simulink subsystem "SMC_mathmatical"  (R2023a)
settings: Solver=VariableStepAuto  StartTime=0.0  StopTime=10.0  RelTol=1e-3

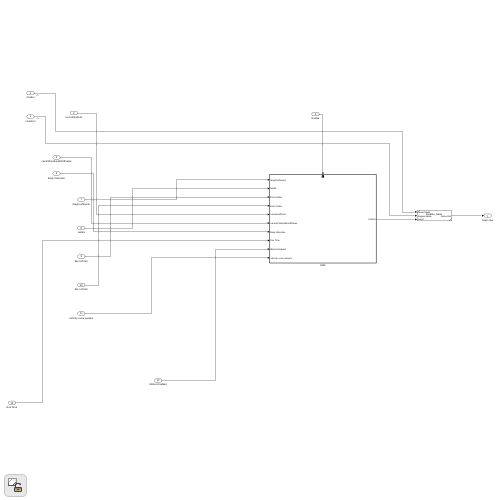
[thumbnail: Simulink's stored preview of the top-level diagram]
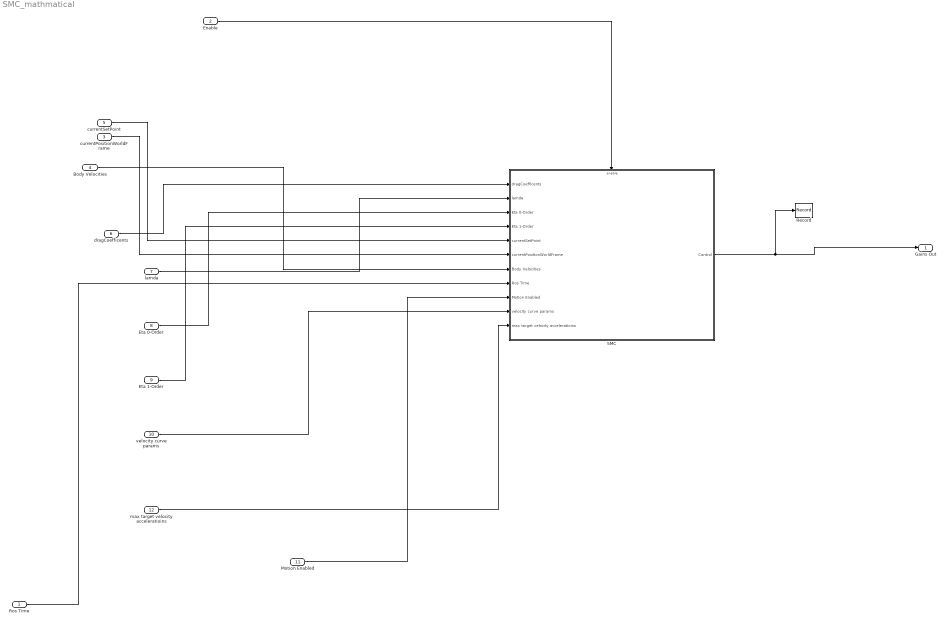
== system SMC_mathmatical ==
  Ros Time : Inport
  Enable : Inport  Port=2
  currentPositionWorldFrame : Inport  Port=3
  Body Velocities : Inport  Port=4
  currentSetPoint : Inport  Port=5
  dragCoefficents : Inport  Port=6
  lamda : Inport  Port=7
  Eta 0-Order : Inport  Port=8
  Eta 1-Order : Inport  Port=9
  velocity curve params : Inport  Port=10
  Motion Enabled : Inport  Port=11
  max target velocity acceleratioins : Inport  Port=12
  Record : Record  FileSettingsInternal="{\"entries\":[{\"content\":{\"excelSettings\":{\"content\":{},\"type\":\"Streamout.ExcelSettings\"}},\"type\":\"Streamout.FileSettingStorage\",\"uuid\":\"\"}],\"packageUris\":[\"http:\\/\\/schema.mathworks.com\\/mf0\\/streamout_blocks\\/R2020a\"],\"version\":\"1.0\"}"  Layout=[1 1]  SignalsInternal="{\"entries\":[{\"content\":{\"signals\":[{\"content\":{\"blockPath\":[],\"dimensions\":[6],\"domain\":\"\",\"hasChildren\":true,\"lineColor\":\"#22b573\",\"port\":1,\"signalID\":150872,\"signalName\":\"SMC\"},\"type\":\"RecordBlkView.Signal\",\"uuid\":\"\"},{\"content\":{\"blockPath\":[],\"channel\":[1],\"dimensions\":[6],\"domain\":\"\",\"lineColor\":\"#0072bd\",\"parentID\":150872,\"plots\":[1],\"port\":1,\"signalID\":150873,\"signalName\":\"SMC\"},\"type\":\"Rec ...(+1177 chars)"  VisualizationBindings="{\"sparklinesplugin\":{\"info\":[{\"bindingParametersList\":[],\"subplotID\":1}]}}"
  SMC : Subsystem
  Gains Out : Outport
  wires:
  SMC/1(Control) -> Gains Out/1, Record/1
  Eta 1-Order/1 -> SMC/4(Eta 1-Order)
  Body Velocities/1 -> SMC/7(Body Velocities)
  Motion Enabled/1 -> SMC/9(Motion Enabled)
  currentPositionWorldFrame/1 -> SMC/6(currentPositionWorldFrame)
  dragCoefficents/1 -> SMC/1(dragCoefficents)
  velocity curve params/1 -> SMC/10(velocity curve params)
  currentSetPoint/1 -> SMC/5(currentSetPoint)
  Enable/1 -> SMC/Enable
  Ros Time/1 -> SMC/8(Ros Time)
  lamda/1 -> SMC/2(lamda)
  Eta 0-Order/1 -> SMC/3(Eta 0-Order)
  max target velocity acceleratioins/1 -> SMC/11(max target velocity acceleratioins)

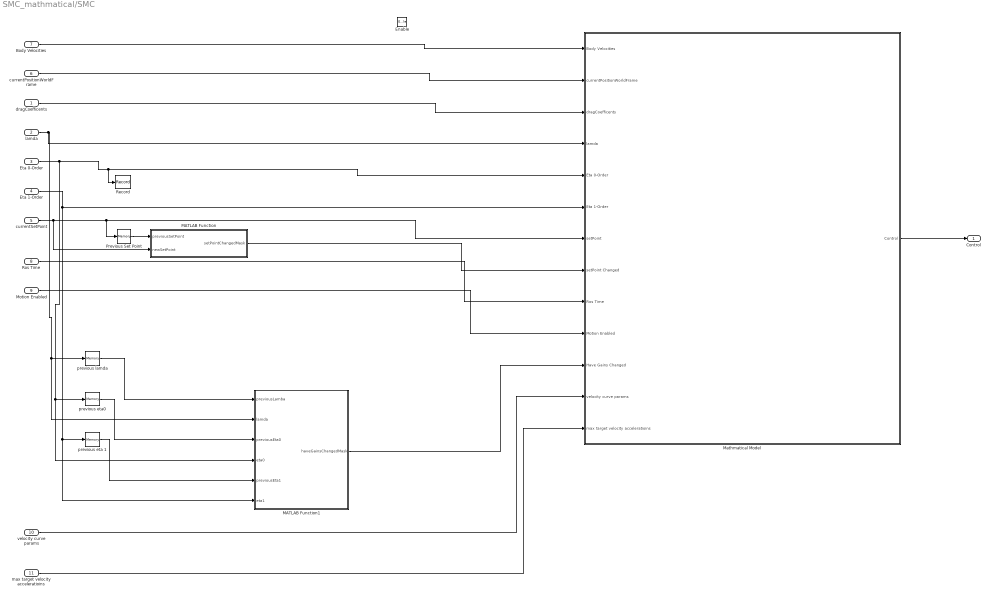
== system SMC_mathmatical/SMC ==
  dragCoefficents : Inport
  lamda : Inport  Port=2
  Eta 0-Order : Inport  Port=3
  Eta 1-Order : Inport  Port=4
  currentSetPoint : Inport  Port=5
  currentPositionWorldFrame : Inport  Port=6
  Body Velocities : Inport  Port=7
  Ros Time : Inport  Port=8
  Motion Enabled : Inport  Port=9
  velocity curve params : Inport  Port=10
  max target velocity acceleratioins : Inport  Port=11
  Enable : EnablePort
  MATLAB Function : MATLAB Function  TreatAsAtomicUnit=on
  MATLAB Function1 : MATLAB Function  TreatAsAtomicUnit=on
  Mathmatical Model : Subsystem
  Previous Set Point : Memory  InitialCondition=[0,0,0,0,0,0,0]  InheritSampleTime=on
  Record : Record  FileSettingsInternal="{\"entries\":[{\"content\":{\"excelSettings\":{\"content\":{},\"type\":\"Streamout.ExcelSettings\"}},\"type\":\"Streamout.FileSettingStorage\",\"uuid\":\"\"}],\"packageUris\":[\"http:\\/\\/schema.mathworks.com\\/mf0\\/streamout_blocks\\/R2020a\"],\"version\":\"1.0\"}"  Layout=[1 1]  SignalsInternal="{\"entries\":[{\"content\":{\"signals\":[{\"content\":{\"blockPath\":[],\"dimensions\":[1,6],\"domain\":\"\",\"hasChildren\":true,\"lineColor\":\"#139fff\",\"port\":1,\"signalID\":151262,\"signalName\":\"Eta 0-Order\"},\"type\":\"RecordBlkView.Signal\",\"uuid\":\"\"},{\"content\":{\"blockPath\":[],\"channel\":[1,1],\"dimensions\":[1,6],\"domain\":\"\",\"lineColor\":\"#edb120\",\"parentID\":151262,\"port\":1,\"signalID\":151263,\"signalName\":\"Eta 0-Order\"},\" ...(+1247 chars)"  VisualizationBindings="{\"sparklinesplugin\":{\"info\":[{\"bindingParametersList\":[],\"subplotID\":1}]}}"
  previous eta 1 : Memory  InheritSampleTime=on
  previous eta0 : Memory  InheritSampleTime=on
  previous lamda : Memory  InheritSampleTime=on
  Control : Outport
  wires:
  max target velocity acceleratioins/1 -> Mathmatical Model/13(max target velocity acceleratioins)
  velocity curve params/1 -> Mathmatical Model/12(velocity curve params)
  MATLAB Function1/1(haveGainsChangedMask) -> Mathmatical Model/11(Have Gains Changed)
  Eta 1-Order/1 -> Mathmatical Model/6(Eta 1-Order), MATLAB Function1/6(eta1), previous eta 1/1
  Eta 0-Order/1 -> MATLAB Function1/4(eta0), previous eta0/1, Mathmatical Model/5(Eta 0-Order), Record/1
  lamda/1 -> previous lamda/1, MATLAB Function1/2(lamda), Mathmatical Model/4(lamda)
  previous eta 1/1 -> MATLAB Function1/5(previousEta1)
  previous eta0/1 -> MATLAB Function1/3(previousEta0)
  previous lamda/1 -> MATLAB Function1/1(previousLamba)
  Motion Enabled/1 -> Mathmatical Model/10(Motion Enabled)
  Ros Time/1 -> Mathmatical Model/9(Ros Time)
  Previous Set Point/1 -> MATLAB Function/1(previousSetPoint)
  MATLAB Function/1(setPointChangedMask) -> Mathmatical Model/8(setPoint Changed)
  Body Velocities/1 -> Mathmatical Model/1(Body Velocities)
  currentPositionWorldFrame/1 -> Mathmatical Model/2(currentPositionWorldFrame)
  currentSetPoint/1 -> Mathmatical Model/7(setPoint), Previous Set Point/1, MATLAB Function/2(newSetPoint)
  Mathmatical Model/1(Control) -> Control/1
  dragCoefficents/1 -> Mathmatical Model/3(dragCoefficents)

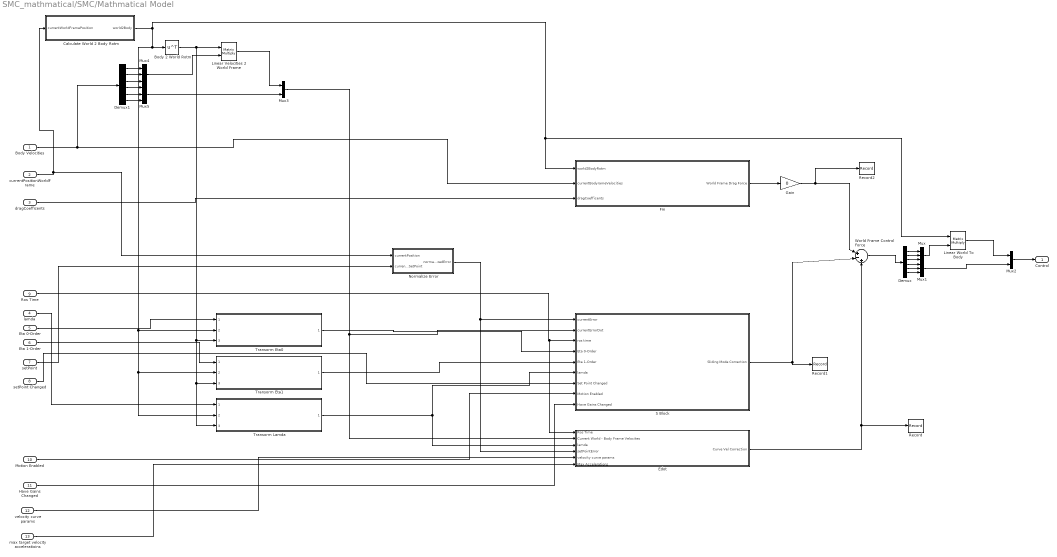
== system SMC_mathmatical/SMC/Mathmatical Model ==
  Body Velocities : Inport
  currentPositionWorldFrame : Inport  Port=2
  dragCoefficents : Inport  Port=3
  lamda : Inport  Port=4
  Eta 0-Order : Inport  Port=5
  Eta 1-Order : Inport  Port=6
  setPoint : Inport  Port=7
  setPoint Changed : Inport  Port=8
  Ros Time : Inport  Port=9
  Motion Enabled : Inport  Port=10
  Have Gains Changed : Inport  Port=11
  velocity curve params : Inport  Port=12
  max target velocity acceleratioins : Inport  Port=13
  Body 2 World Rotm : Math  Operator=transpose
  Calculate World 2 Body Rotm : MATLAB Function  TreatAsAtomicUnit=on
  Demux : Demux  Outputs=6
  Demux1 : Demux  Outputs=6
  Edot : Subsystem
  Fm : Subsystem
  Gain : Gain  Gain=0
  Linear Velocities 2 World Frame : Product  Multiplication=Matrix(*)
  Linear World To Body : Product  Multiplication=Matrix(*)
  Mux{,1,4..5} (4 alike) : Mux  Inputs=3
  Mux2 : Mux  Inputs=2
  Mux3 : Mux  Inputs=2
  Normalize Error : MATLAB Function  TreatAsAtomicUnit=on
  Record : Record  FileSettingsInternal="{\"entries\":[{\"content\":{\"excelSettings\":{\"content\":{},\"type\":\"Streamout.ExcelSettings\"}},\"type\":\"Streamout.FileSettingStorage\",\"uuid\":\"\"}],\"packageUris\":[\"http:\\/\\/schema.mathworks.com\\/mf0\\/streamout_blocks\\/R2020a\"],\"version\":\"1.0\"}"  Layout=[1 1]  SignalsInternal="{\"entries\":[{\"content\":{\"signals\":[{\"content\":{\"blockPath\":[],\"dimensions\":[6,1],\"domain\":\"\",\"hasChildren\":true,\"lineColor\":\"#ff6929\",\"port\":1,\"signalID\":150991,\"signalName\":\"Edot\"},\"type\":\"RecordBlkView.Signal\",\"uuid\":\"\"},{\"content\":{\"blockPath\":[],\"channel\":[1,1],\"dimensions\":[6,1],\"domain\":\"\",\"lineColor\":\"#4dbeee\",\"parentID\":150991,\"plots\":[1],\"port\":1,\"signalID\":150992,\"signalName\":\"Edot\"},\"ty ...(+1210 chars)"  VisualizationBindings="{\"sparklinesplugin\":{\"info\":[{\"bindingParametersList\":[],\"subplotID\":1}]}}"
  Record1 : Record  FileSettingsInternal="{\"entries\":[{\"content\":{\"excelSettings\":{\"content\":{},\"type\":\"Streamout.ExcelSettings\"}},\"type\":\"Streamout.FileSettingStorage\",\"uuid\":\"\"}],\"packageUris\":[\"http:\\/\\/schema.mathworks.com\\/mf0\\/streamout_blocks\\/R2020a\"],\"version\":\"1.0\"}"  Layout=[1 1]  SignalsInternal="{\"entries\":[{\"content\":{\"signals\":[{\"content\":{\"blockPath\":[],\"dimensions\":[6,1],\"domain\":\"\",\"hasChildren\":true,\"lineColor\":\"#fe330a\",\"port\":1,\"signalID\":151008,\"signalName\":\"S Block\"},\"type\":\"RecordBlkView.Signal\",\"uuid\":\"\"},{\"content\":{\"blockPath\":[],\"channel\":[1,1],\"dimensions\":[6,1],\"domain\":\"\",\"lineColor\":\"#0072bd\",\"parentID\":151008,\"plots\":[1],\"port\":1,\"signalID\":151009,\"signalName\":\"S Block ...(+1231 chars)"  VisualizationBindings="{\"sparklinesplugin\":{\"info\":[{\"bindingParametersList\":[],\"subplotID\":1}]}}"
  Record2 : Record  FileSettingsInternal="{\"entries\":[{\"content\":{\"excelSettings\":{\"content\":{},\"type\":\"Streamout.ExcelSettings\"}},\"type\":\"Streamout.FileSettingStorage\",\"uuid\":\"\"}],\"packageUris\":[\"http:\\/\\/schema.mathworks.com\\/mf0\\/streamout_blocks\\/R2020a\"],\"version\":\"1.0\"}"  Layout=[1 1]  SignalsInternal="{\"entries\":[{\"content\":{\"signals\":[{\"content\":{\"blockPath\":[],\"dimensions\":[6],\"domain\":\"\",\"hasChildren\":true,\"lineColor\":\"#22b573\",\"port\":1,\"signalID\":151025,\"signalName\":\"Gain\"},\"type\":\"RecordBlkView.Signal\",\"uuid\":\"\"},{\"content\":{\"blockPath\":[],\"channel\":[1],\"dimensions\":[6],\"domain\":\"\",\"lineColor\":\"#edb120\",\"parentID\":151025,\"plots\":[1],\"port\":1,\"signalID\":151026,\"signalName\":\"Gain\"},\"type\":\"R ...(+1232 chars)"  VisualizationBindings="{\"sparklinesplugin\":{\"info\":[{\"bindingParametersList\":[],\"subplotID\":1}]}}"
  S Block : Subsystem
  Transorm Eta0 : Subsystem  ReferencedSubsystem=Tranfsform_Linear_Gains_To_World
  Transorm Eta1 : Subsystem  ReferencedSubsystem=Tranfsform_Linear_Gains_To_World
  Transorm Lamda : Subsystem  ReferencedSubsystem=Tranfsform_Linear_Gains_To_World
  World Frame Control Force : Sum  Inputs=|+-+
  Control : Outport
  wires:
  max target velocity acceleratioins/1 -> Edot/6(Max Accelerations)
  velocity curve params/1 -> Edot/5(velocity curve params)
  Have Gains Changed/1 -> S Block/9(Have Gains Changed)
  Motion Enabled/1 -> S Block/8(Motion Enabled)
  Transorm Eta0/1 -> S Block/4(Eta 0-Order)
  Body 2 World Rotm/1 -> Linear Velocities 2 World Frame/1, Transorm Eta0/3, Transorm Eta1/3, Transorm Lamda/3
  Edot/1(Curve Vel Correction) -> World Frame Control Force/3, Record/1
  Gain/1 -> World Frame Control Force/1, Record2/1
  Eta 1-Order/1 -> Transorm Eta1/1
  setPoint/1 -> Normalize Error/2(currentSetPoint)
  Normalize Error/1(normalizedError) -> S Block/1(currentError), Edot/4(setPointError)
  Ros Time/1 -> S Block/3(ros time), Edot/1(Ros Time)
  setPoint Changed/1 -> S Block/7(Set Point Changed)
  Mux3/1 -> Edot/2(Current World - Body Frame Velocites), S Block/2(currentErrorDot)
  Eta 0-Order/1 -> Transorm Eta0/1
  lamda/1 -> Transorm Lamda/1
  Transorm Eta1/1 -> S Block/5(Eta 1-Order)
  Transorm Lamda/1 -> Edot/3(lamda), S Block/6(lamda)
  Mux5/1 -> Mux3/2
  Fm/1(World Frame Drag Force) -> Gain/1
  Demux1/6 -> Mux5/3
  Demux1/4 -> Mux5/1
  Demux1/5 -> Mux5/2
  Demux1/3 -> Mux4/3
  Demux1/1 -> Mux4/1
  Demux1/2 -> Mux4/2
  Mux4/1 -> Linear Velocities 2 World Frame/2
  Linear Velocities 2 World Frame/1 -> Mux3/1
  dragCoefficents/1 -> Fm/3(dragCoefficents)
  Calculate World 2 Body Rotm/1(world2Body) -> Fm/1(world2BodyRotm), Linear World To Body/1, Transorm Lamda/2, Transorm Eta1/2, Transorm Eta0/2, Body 2 World Rotm/1
  Mux2/1 -> Control/1
  Mux1/1 -> Mux2/2
  Linear World To Body/1 -> Mux2/1
  Mux/1 -> Linear World To Body/2
  Demux/4 -> Mux1/1
  Demux/5 -> Mux1/2
  Demux/6 -> Mux1/3
  Demux/3 -> Mux/3
  Demux/2 -> Mux/2
  Demux/1 -> Mux/1
  World Frame Control Force/1 -> Demux/1
  S Block/1("Sliding Mode Correction ") -> Record1/1, World Frame Control Force/2
  currentPositionWorldFrame/1 -> Calculate World 2 Body Rotm/1(currentWorldFramePosition), Normalize Error/1(currentPosition)
  Body Velocities/1 -> Demux1/1, Fm/2(currentBodyrameVelocities)

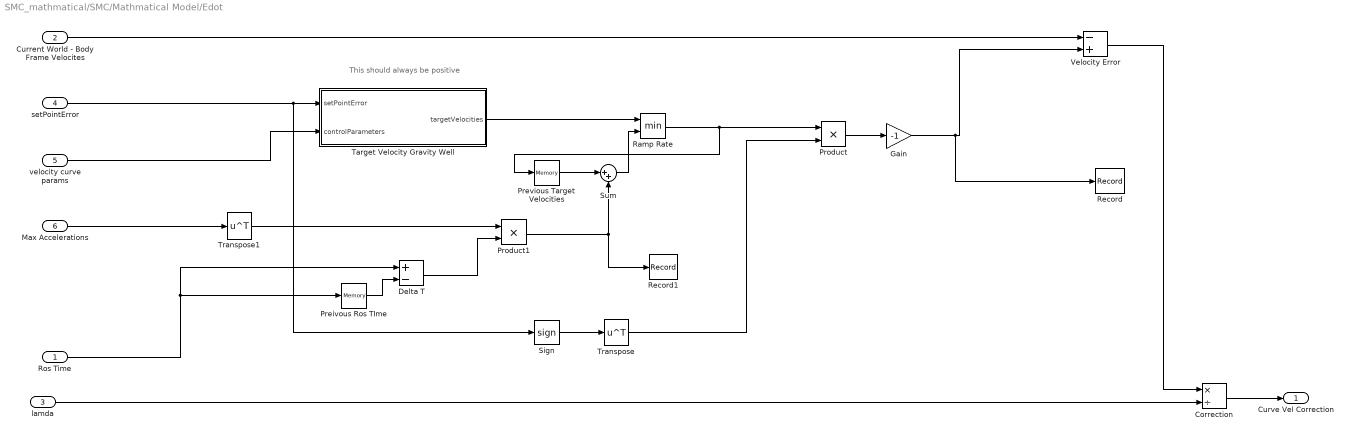
== system SMC_mathmatical/SMC/Mathmatical Model/Edot ==
  note: This should always be positive
  Ros Time : Inport
  Current World - Body Frame Velocites : Inport  Port=2
  lamda : Inport  Port=3
  setPointError : Inport  Port=4
  velocity curve params : Inport  Port=5
  Max Accelerations : Inport  Port=6
  Correction : Product  Inputs=*/
  Delta T : Sum  Inputs=+-
  Gain : Gain  Gain=-1
  Preivous Ros TIme : Memory
  Previous Target Velocities : Memory
  Product : Product
  Product1 : Product
  Ramp Rate : MinMax  Inputs=2
  Record : Record  FileSettingsInternal="{\"entries\":[{\"content\":{\"excelSettings\":{\"content\":{},\"type\":\"Streamout.ExcelSettings\"}},\"type\":\"Streamout.FileSettingStorage\",\"uuid\":\"\"}],\"packageUris\":[\"http:\\/\\/schema.mathworks.com\\/mf0\\/streamout_blocks\\/R2020a\"],\"version\":\"1.0\"}"  Layout=[1 1]  SignalsInternal="{\"entries\":[{\"content\":{\"signals\":[{\"content\":{\"blockPath\":[],\"dimensions\":[6,1],\"domain\":\"\",\"hasChildren\":true,\"lineColor\":\"#edb120\",\"port\":1,\"signalID\":150889,\"signalName\":\"Product\"},\"type\":\"RecordBlkView.Signal\",\"uuid\":\"\"},{\"content\":{\"blockPath\":[],\"channel\":[1,1],\"dimensions\":[6,1],\"domain\":\"\",\"lineColor\":\"#7e2f8e\",\"parentID\":150889,\"plots\":[1],\"port\":1,\"signalID\":150890,\"signalName\":\"Product ...(+1231 chars)"  VisualizationBindings="{\"sparklinesplugin\":{\"info\":[{\"bindingParametersList\":[],\"subplotID\":1}]}}"
  Record1 : Record  FileSettingsInternal="{\"entries\":[{\"content\":{\"excelSettings\":{\"content\":{},\"type\":\"Streamout.ExcelSettings\"}},\"type\":\"Streamout.FileSettingStorage\",\"uuid\":\"\"}],\"packageUris\":[\"http:\\/\\/schema.mathworks.com\\/mf0\\/streamout_blocks\\/R2020a\"],\"version\":\"1.0\"}"  Layout=[1 1]  SignalsInternal="{\"entries\":[{\"content\":{\"signals\":[{\"content\":{\"blockPath\":[],\"dimensions\":[6,1],\"domain\":\"\",\"hasChildren\":true,\"lineColor\":\"#ff6929\",\"port\":1,\"signalID\":150906,\"signalName\":\"Product1\"},\"type\":\"RecordBlkView.Signal\",\"uuid\":\"\"},{\"content\":{\"blockPath\":[],\"channel\":[1,1],\"dimensions\":[6,1],\"domain\":\"\",\"lineColor\":\"#b746ff\",\"parentID\":150906,\"plots\":[1],\"port\":1,\"signalID\":150907,\"signalName\":\"Produc ...(+1238 chars)"  VisualizationBindings="{\"sparklinesplugin\":{\"info\":[{\"bindingParametersList\":[],\"subplotID\":1}]}}"
  Sign : Signum
  Sum : Sum  Inputs=|++
  Target Velocity Gravity Well : MATLAB Function  TreatAsAtomicUnit=on
  Transpose : Math  Operator=transpose
  Transpose1 : Math  Operator=transpose
  Velocity Error : Sum  Inputs=-+
  Curve Vel Correction : Outport
  wires:
  Gain/1 -> Velocity Error/2, Record/1
  Transpose1/1 -> Product1/1
  Max Accelerations/1 -> Transpose1/1
  Product1/1 -> Sum/2, Record1/1
  Transpose/1 -> Product/2
  Delta T/1 -> Product1/2
  Ros Time/1 -> Preivous Ros TIme/1, Delta T/1
  Preivous Ros TIme/1 -> Delta T/2
  Sign/1 -> Transpose/1
  Product/1 -> Gain/1
  Ramp Rate/1 -> Product/1, Previous Target Velocities/1
  Previous Target Velocities/1 -> Sum/1
  Sum/1 -> Ramp Rate/2
  velocity curve params/1 -> Target Velocity Gravity Well/2(controlParameters)
  Target Velocity Gravity Well/1(targetVelocities) -> Ramp Rate/1
  setPointError/1 -> Target Velocity Gravity Well/1(setPointError), Sign/1
  Velocity Error/1 -> Correction/1
  Current World - Body Frame Velocites/1 -> Velocity Error/1
  lamda/1 -> Correction/2
  Correction/1 -> Curve Vel Correction/1

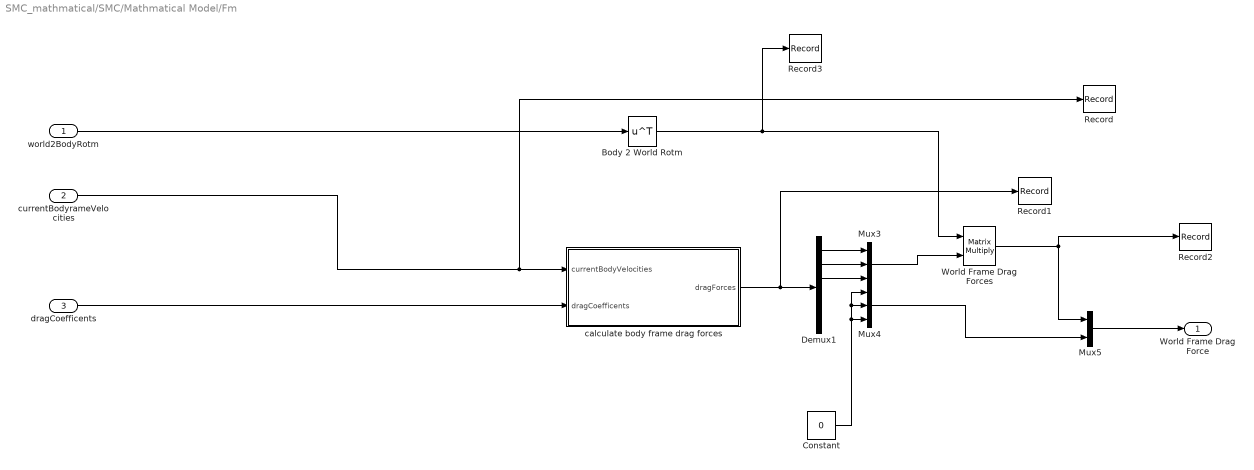
== system SMC_mathmatical/SMC/Mathmatical Model/Fm ==
  world2BodyRotm : Inport
  currentBodyrameVelocities : Inport  Port=2
  dragCoefficents : Inport  Port=3
  Body 2 World Rotm : Math  Operator=transpose
  Constant : Constant  Value=0
  Demux1 : Demux  Outputs=6
  Mux3 : Mux  Inputs=3
  Mux4 : Mux  Inputs=3
  Mux5 : Mux  Inputs=2
  Record : Record  FileSettingsInternal="{\"entries\":[{\"content\":{\"excelSettings\":{\"content\":{},\"type\":\"Streamout.ExcelSettings\"}},\"type\":\"Streamout.FileSettingStorage\",\"uuid\":\"\"}],\"packageUris\":[\"http:\\/\\/schema.mathworks.com\\/mf0\\/streamout_blocks\\/R2020a\"],\"version\":\"1.0\"}"  Layout=[1 1]  SignalsInternal="{\"entries\":[{\"content\":{\"signals\":[{\"content\":{\"blockPath\":[],\"dimensions\":[6],\"domain\":\"\",\"hasChildren\":true,\"lineColor\":\"#d95319\",\"port\":1,\"signalID\":150923,\"signalName\":\"currentBodyrameVelocities\"},\"type\":\"RecordBlkView.Signal\",\"uuid\":\"\"},{\"content\":{\"blockPath\":[],\"channel\":[1],\"dimensions\":[6],\"domain\":\"\",\"lineColor\":\"#b746ff\",\"parentID\":150923,\"plots\":[1],\"port\":1,\"signalID\":150924,\"signalNa ...(+1367 chars)"  VisualizationBindings="{\"sparklinesplugin\":{\"info\":[{\"bindingParametersList\":[],\"subplotID\":1}]}}"
  Record1 : Record  FileSettingsInternal="{\"entries\":[{\"content\":{\"excelSettings\":{\"content\":{},\"type\":\"Streamout.ExcelSettings\"}},\"type\":\"Streamout.FileSettingStorage\",\"uuid\":\"\"}],\"packageUris\":[\"http:\\/\\/schema.mathworks.com\\/mf0\\/streamout_blocks\\/R2020a\"],\"version\":\"1.0\"}"  Layout=[1 1]  SignalsInternal="{\"entries\":[{\"content\":{\"signals\":[{\"content\":{\"blockPath\":[],\"dimensions\":[6,1],\"domain\":\"\",\"hasChildren\":true,\"lineColor\":\"#7e2f8e\",\"port\":1,\"signalID\":150940,\"signalName\":\"calculate body frame drag forces\"},\"type\":\"RecordBlkView.Signal\",\"uuid\":\"\"},{\"content\":{\"blockPath\":[],\"channel\":[1,1],\"dimensions\":[6,1],\"domain\":\"\",\"lineColor\":\"#139fff\",\"parentID\":150940,\"plots\":[1],\"port\":1,\"signalID\":150 ...(+1454 chars)"  VisualizationBindings="{\"sparklinesplugin\":{\"info\":[{\"bindingParametersList\":[],\"subplotID\":1}]}}"
  Record2 : Record  FileSettingsInternal="{\"entries\":[{\"content\":{\"excelSettings\":{\"content\":{},\"type\":\"Streamout.ExcelSettings\"}},\"type\":\"Streamout.FileSettingStorage\",\"uuid\":\"\"}],\"packageUris\":[\"http:\\/\\/schema.mathworks.com\\/mf0\\/streamout_blocks\\/R2020a\"],\"version\":\"1.0\"}"  SignalsInternal="{\"entries\":[{\"content\":{\"signals\":[{\"content\":{\"blockPath\":[],\"dimensions\":[3],\"domain\":\"\",\"hasChildren\":true,\"lineColor\":\"#4dbeee\",\"port\":1,\"signalID\":150957,\"signalName\":\"World Frame Drag Forces\"},\"type\":\"RecordBlkView.Signal\",\"uuid\":\"\"},{\"content\":{\"blockPath\":[],\"channel\":[1],\"dimensions\":[3],\"domain\":\"\",\"lineColor\":\"#b746ff\",\"parentID\":150957,\"plots\":[1],\"port\":1,\"signalID\":150958,\"signalName ...(+675 chars)"  VisualizationBindings="{\"sparklinesplugin\":{\"info\":[{\"bindingParametersList\":[],\"subplotID\":1}]}}"
  Record3 : Record  FileSettingsInternal="{\"entries\":[{\"content\":{\"excelSettings\":{\"content\":{},\"type\":\"Streamout.ExcelSettings\"}},\"type\":\"Streamout.FileSettingStorage\",\"uuid\":\"\"}],\"packageUris\":[\"http:\\/\\/schema.mathworks.com\\/mf0\\/streamout_blocks\\/R2020a\"],\"version\":\"1.0\"}"  Layout=[1 1]  SignalsInternal="{\"entries\":[{\"content\":{\"signals\":[{\"content\":{\"blockPath\":[],\"dimensions\":[3,3],\"domain\":\"\",\"hasChildren\":true,\"lineColor\":\"#139fff\",\"port\":1,\"signalID\":150968,\"signalName\":\"Body 2 World Rotm\"},\"type\":\"RecordBlkView.Signal\",\"uuid\":\"\"},{\"content\":{\"blockPath\":[],\"channel\":[1,1],\"dimensions\":[3,3],\"domain\":\"\",\"lineColor\":\"#a2142f\",\"parentID\":150968,\"plots\":[1],\"port\":1,\"signalID\":150969,\"signalName ...(+2033 chars)"  VisualizationBindings="{\"sparklinesplugin\":{\"info\":[{\"bindingParametersList\":[],\"subplotID\":1}]}}"
  World Frame Drag Forces : Product  Multiplication=Matrix(*)
  calculate body frame drag forces : MATLAB Function  TreatAsAtomicUnit=on
  World Frame Drag Force : Outport
  wires:
  Constant/1 -> Mux4/1, Mux4/2, Mux4/3
  Mux4/1 -> Mux5/2
  calculate body frame drag forces/1(dragForces) -> Demux1/1, Record1/1
  Body 2 World Rotm/1 -> World Frame Drag Forces/1, Record3/1
  world2BodyRotm/1 -> Body 2 World Rotm/1
  dragCoefficents/1 -> calculate body frame drag forces/2(dragCoefficents)
  currentBodyrameVelocities/1 -> calculate body frame drag forces/1(currentBodyVelocities), Record/1
  Demux1/2 -> Mux3/2
  Mux5/1 -> World Frame Drag Force/1
  Demux1/3 -> Mux3/3
  Mux3/1 -> World Frame Drag Forces/2
  Demux1/1 -> Mux3/1
  World Frame Drag Forces/1 -> Record2/1, Mux5/1

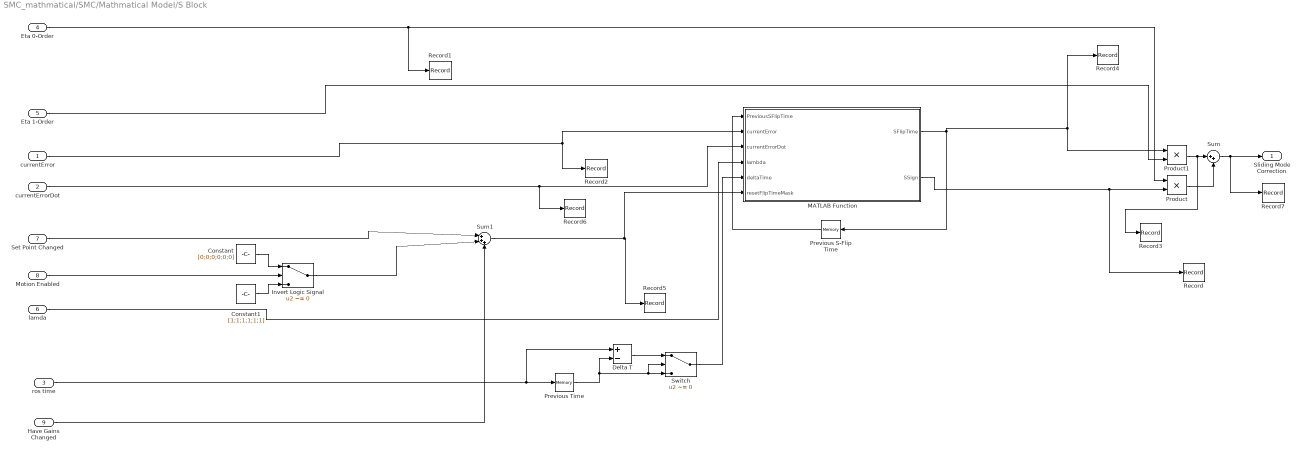
== system SMC_mathmatical/SMC/Mathmatical Model/S Block ==
  currentError : Inport
  currentErrorDot : Inport  Port=2
  ros time : Inport  Port=3
  Eta 0-Order : Inport  Port=4
  Eta 1-Order : Inport  Port=5
  lamda : Inport  Port=6
  Set Point Changed : Inport  Port=7
  Motion Enabled : Inport  Port=8
  Have Gains Changed : Inport  Port=9
  Constant : Constant  Value=[0;0;0;0;0;0]
  Constant1 : Constant  Value=[1;1;1;1;1;1]
  Delta T : Sum  Inputs=+-
  Invert Logic Signal : Switch  Criteria=u2 ~= 0  SaturateOnIntegerOverflow=off  InputSameDT=off
  MATLAB Function : MATLAB Function  TreatAsAtomicUnit=on
  Previous S-Flip Time : Memory  InitialCondition=[0;0;0;0;0;0]  InheritSampleTime=on
  Previous Time : Memory  InheritSampleTime=on
  Product : Product
  Product1 : Product
  Record : Record  FileSettingsInternal="{\"entries\":[{\"content\":{\"excelSettings\":{\"content\":{},\"type\":\"Streamout.ExcelSettings\"}},\"type\":\"Streamout.FileSettingStorage\",\"uuid\":\"\"}],\"packageUris\":[\"http:\\/\\/schema.mathworks.com\\/mf0\\/streamout_blocks\\/R2020a\"],\"version\":\"1.0\"}"  Layout=[1 1]  SignalsInternal="{\"entries\":[{\"content\":{\"signals\":[{\"content\":{\"blockPath\":[],\"dimensions\":[6,1],\"domain\":\"\",\"hasChildren\":true,\"lineColor\":\"#b746ff\",\"port\":1,\"signalID\":151042,\"signalName\":\"MATLAB Function:2\"},\"type\":\"RecordBlkView.Signal\",\"uuid\":\"\"},{\"content\":{\"blockPath\":[],\"channel\":[1,1],\"dimensions\":[6,1],\"domain\":\"\",\"lineColor\":\"#77ac30\",\"parentID\":151042,\"plots\":[1],\"port\":1,\"signalID\":151043,\"signalName ...(+1313 chars)"  VisualizationBindings="{\"sparklinesplugin\":{\"info\":[{\"bindingParametersList\":[],\"subplotID\":1}]}}"
  Record1 : Record  FileSettingsInternal="{\"entries\":[{\"content\":{\"excelSettings\":{\"content\":{},\"type\":\"Streamout.ExcelSettings\"}},\"type\":\"Streamout.FileSettingStorage\",\"uuid\":\"\"}],\"packageUris\":[\"http:\\/\\/schema.mathworks.com\\/mf0\\/streamout_blocks\\/R2020a\"],\"version\":\"1.0\"}"  Layout=[1 1]  SignalsInternal="{\"entries\":[{\"content\":{\"signals\":[{\"content\":{\"blockPath\":[],\"dimensions\":[6],\"domain\":\"\",\"hasChildren\":true,\"lineColor\":\"#ff13a6\",\"port\":1,\"signalID\":151059,\"signalName\":\"Eta 0-Order\"},\"type\":\"RecordBlkView.Signal\",\"uuid\":\"\"},{\"content\":{\"blockPath\":[],\"channel\":[1],\"dimensions\":[6],\"domain\":\"\",\"lineColor\":\"#ff6929\",\"parentID\":151059,\"port\":1,\"signalID\":151060,\"signalName\":\"Eta 0-Order\"},\"type\": ...(+1221 chars)"  VisualizationBindings="{\"sparklinesplugin\":{\"info\":[{\"bindingParametersList\":[],\"subplotID\":1}]}}"
  Record2 : Record  FileSettingsInternal="{\"entries\":[{\"content\":{\"excelSettings\":{\"content\":{},\"type\":\"Streamout.ExcelSettings\"}},\"type\":\"Streamout.FileSettingStorage\",\"uuid\":\"\"}],\"packageUris\":[\"http:\\/\\/schema.mathworks.com\\/mf0\\/streamout_blocks\\/R2020a\"],\"version\":\"1.0\"}"  Layout=[1 1]  SignalsInternal="{\"entries\":[{\"content\":{\"signals\":[{\"content\":{\"blockPath\":[],\"dimensions\":[1,6],\"domain\":\"\",\"hasChildren\":true,\"lineColor\":\"#22b573\",\"port\":1,\"signalID\":151076,\"signalName\":\"currentError\"},\"type\":\"RecordBlkView.Signal\",\"uuid\":\"\"},{\"content\":{\"blockPath\":[],\"channel\":[1,1],\"dimensions\":[1,6],\"domain\":\"\",\"lineColor\":\"#7e2f8e\",\"parentID\":151076,\"port\":1,\"signalID\":151077,\"signalName\":\"currentError\"} ...(+1254 chars)"  VisualizationBindings="{\"sparklinesplugin\":{\"info\":[{\"bindingParametersList\":[],\"subplotID\":1}]}}"
  Record3 : Record  FileSettingsInternal="{\"entries\":[{\"content\":{\"excelSettings\":{\"content\":{},\"type\":\"Streamout.ExcelSettings\"}},\"type\":\"Streamout.FileSettingStorage\",\"uuid\":\"\"}],\"packageUris\":[\"http:\\/\\/schema.mathworks.com\\/mf0\\/streamout_blocks\\/R2020a\"],\"version\":\"1.0\"}"  Layout=[1 1]  SignalsInternal="{\"entries\":[{\"content\":{\"signals\":[{\"content\":{\"blockPath\":[],\"dimensions\":[6,1],\"domain\":\"\",\"hasChildren\":true,\"lineColor\":\"#d95319\",\"port\":1,\"signalID\":151093,\"signalName\":\"Product1\"},\"type\":\"RecordBlkView.Signal\",\"uuid\":\"\"},{\"content\":{\"blockPath\":[],\"channel\":[1,1],\"dimensions\":[6,1],\"domain\":\"\",\"lineColor\":\"#b746ff\",\"parentID\":151093,\"plots\":[1],\"port\":1,\"signalID\":151094,\"signalName\":\"Produc ...(+1250 chars)"  VisualizationBindings="{\"sparklinesplugin\":{\"info\":[{\"bindingParametersList\":[],\"subplotID\":1}]}}"
  Record4 : Record  FileSettingsInternal="{\"entries\":[{\"content\":{\"excelSettings\":{\"content\":{},\"type\":\"Streamout.ExcelSettings\"}},\"type\":\"Streamout.FileSettingStorage\",\"uuid\":\"\"}],\"packageUris\":[\"http:\\/\\/schema.mathworks.com\\/mf0\\/streamout_blocks\\/R2020a\"],\"version\":\"1.0\"}"  Layout=[1 1]  SignalsInternal="{\"entries\":[{\"content\":{\"signals\":[{\"content\":{\"blockPath\":[],\"dimensions\":[6,1],\"domain\":\"\",\"hasChildren\":true,\"lineColor\":\"#7e2f8e\",\"port\":1,\"signalID\":151110,\"signalName\":\"MATLAB Function:1\"},\"type\":\"RecordBlkView.Signal\",\"uuid\":\"\"},{\"content\":{\"blockPath\":[],\"channel\":[1,1],\"dimensions\":[6,1],\"domain\":\"\",\"lineColor\":\"#4dbeee\",\"parentID\":151110,\"plots\":[1],\"port\":1,\"signalID\":151111,\"signalName ...(+1301 chars)"  VisualizationBindings="{\"sparklinesplugin\":{\"info\":[{\"bindingParametersList\":[],\"subplotID\":1}]}}"
  Record5 : Record  FileSettingsInternal="{\"entries\":[{\"content\":{\"excelSettings\":{\"content\":{},\"type\":\"Streamout.ExcelSettings\"}},\"type\":\"Streamout.FileSettingStorage\",\"uuid\":\"\"}],\"packageUris\":[\"http:\\/\\/schema.mathworks.com\\/mf0\\/streamout_blocks\\/R2020a\"],\"version\":\"1.0\"}"  Layout=[1 1]  SignalsInternal="{\"entries\":[{\"content\":{\"signals\":[{\"content\":{\"blockPath\":[],\"dimensions\":[1,6],\"domain\":\"\",\"hasChildren\":true,\"lineColor\":\"#4dbeee\",\"port\":1,\"signalID\":151127,\"signalName\":\"Sum1\"},\"type\":\"RecordBlkView.Signal\",\"uuid\":\"\"},{\"content\":{\"blockPath\":[],\"channel\":[1,1],\"dimensions\":[1,6],\"domain\":\"\",\"lineColor\":\"#ff13a6\",\"parentID\":151127,\"plots\":[1],\"port\":1,\"signalID\":151128,\"signalName\":\"Sum1\"},\"ty ...(+1210 chars)"  VisualizationBindings="{\"sparklinesplugin\":{\"info\":[{\"bindingParametersList\":[],\"subplotID\":1}]}}"
  Record6 : Record  FileSettingsInternal="{\"entries\":[{\"content\":{\"excelSettings\":{\"content\":{},\"type\":\"Streamout.ExcelSettings\"}},\"type\":\"Streamout.FileSettingStorage\",\"uuid\":\"\"}],\"packageUris\":[\"http:\\/\\/schema.mathworks.com\\/mf0\\/streamout_blocks\\/R2020a\"],\"version\":\"1.0\"}"  Layout=[1 1]  SignalsInternal="{\"entries\":[{\"content\":{\"signals\":[{\"content\":{\"blockPath\":[],\"dimensions\":[6],\"domain\":\"\",\"hasChildren\":true,\"lineColor\":\"#139fff\",\"port\":1,\"signalID\":151144,\"signalName\":\"currentErrorDot\"},\"type\":\"RecordBlkView.Signal\",\"uuid\":\"\"},{\"content\":{\"blockPath\":[],\"channel\":[1],\"dimensions\":[6],\"domain\":\"\",\"lineColor\":\"#a2142f\",\"parentID\":151144,\"port\":1,\"signalID\":151145,\"signalName\":\"currentErrorDot\"} ...(+1249 chars)"  VisualizationBindings="{\"sparklinesplugin\":{\"info\":[{\"bindingParametersList\":[],\"subplotID\":1}]}}"
  Record7 : Record  FileSettingsInternal="{\"entries\":[{\"content\":{\"excelSettings\":{\"content\":{},\"type\":\"Streamout.ExcelSettings\"}},\"type\":\"Streamout.FileSettingStorage\",\"uuid\":\"\"}],\"packageUris\":[\"http:\\/\\/schema.mathworks.com\\/mf0\\/streamout_blocks\\/R2020a\"],\"version\":\"1.0\"}"  Layout=[1 1]  SignalsInternal="{\"entries\":[{\"content\":{\"signals\":[{\"content\":{\"blockPath\":[],\"dimensions\":[6,1],\"domain\":\"\",\"hasChildren\":true,\"lineColor\":\"#b746ff\",\"port\":1,\"signalID\":151161,\"signalName\":\"Sum\"},\"type\":\"RecordBlkView.Signal\",\"uuid\":\"\"},{\"content\":{\"blockPath\":[],\"channel\":[1,1],\"dimensions\":[6,1],\"domain\":\"\",\"lineColor\":\"#4dbeee\",\"parentID\":151161,\"port\":1,\"signalID\":151162,\"signalName\":\"Sum\"},\"type\":\"RecordBlk ...(+1191 chars)"  VisualizationBindings="{\"sparklinesplugin\":{\"info\":[{\"bindingParametersList\":[],\"subplotID\":1}]}}"
  Sum : Sum  Inputs=|++
  Sum1 : Sum  Inputs=|+++
  Switch : Switch  Criteria=u2 ~= 0  SaturateOnIntegerOverflow=off  InputSameDT=off
  "Sliding Mode Correction " : Outport
  wires:
  Invert Logic Signal/1 -> Sum1/2
  Have Gains Changed/1 -> Sum1/3
  Delta T/1 -> Switch/1
  Switch/1 -> MATLAB Function/5(deltaTime)
  ros time/1 -> Delta T/1, Previous Time/1
  Previous Time/1 -> Delta T/2, Switch/3, Switch/2
  Constant1/1 -> Invert Logic Signal/3
  Constant/1 -> Invert Logic Signal/1
  Motion Enabled/1 -> Invert Logic Signal/2
  Set Point Changed/1 -> Sum1/1
  Sum1/1 -> Record5/1, MATLAB Function/6(resetFlipTimeMask)
  lamda/1 -> MATLAB Function/4(lambda)
  Eta 1-Order/1 -> Product1/2
  Eta 0-Order/1 -> Product/1, Record1/1
  Previous S-Flip Time/1 -> MATLAB Function/1(PreviousSFlipTime)
  Sum/1 -> Record7/1, "Sliding Mode Correction "/1
  MATLAB Function/1(SFlipTime) -> Previous S-Flip Time/1, Product1/1, Record4/1
  Product1/1 -> Sum/1, Record3/1
  Product/1 -> Sum/2
  currentError/1 -> Record2/1, MATLAB Function/2(currentError)
  currentErrorDot/1 -> MATLAB Function/3(currentErrorDot), Record6/1
  MATLAB Function/2(SSign) -> Product/2, Record/1

== matlab function SMC_mathmatical/SMC/MATLAB Function ==
function setPointChangedMask = fcn(previousSetPoint, newSetPoint)

setPointChangedMask = zeros(1,6);

%determine wether or not the set point has chnaged - element wise

previousEulerSetPoint = [previousSetPoint(1), previousSetPoint(2), previousSetPoint(3), quat2eul([previousSetPoint(7), previousSetPoint(4), previousSetPoint(5), previousSetPoint(6)])];
newEulerSetPoint = [newSetPoint(1), newSetPoint(2), newSetPoint(3), quat2eul([newSetPoint(7), newSetPoint(4), newSetPoint(5), newSetPoint(6)])];

%not changed = 0, true - everything else
setPointChangedMask = abs(previousEulerSetPoint - newEulerSetPoint);

%allow buffer on angular to account for slight shift due to conversion
%error...
for i=4:6
    if(setPointChangedMask(i) < .1)
        setPointChangedMask(i) = 0;
    end

    %catch nans and reset if they occur
    if(isnan(setPointChangedMask(i)))
        setPointChangedMask(i) = 1;
    end
end

== matlab function SMC_mathmatical/SMC/MATLAB Function1 ==
function haveGainsChangedMask = fcn(previousLamba, lamda, previousEta0, eta0, previousEta1, eta1)

%determine wether or not the set point has chnaged element wise
haveGainsChangedMask = abs(previousLamba - lamda) + abs(previousEta0 - eta0) + abs(previousEta1 - eta1);

== matlab function SMC_mathmatical/SMC/Mathmatical Model/Calculate World 2 Body Rotm ==
function world2Body = fcn(currentWorldFramePosition)

%convert ros2 quat to matlab quat - quat is last 
quat = [currentWorldFramePosition(7), currentWorldFramePosition(4), currentWorldFramePosition(5), currentWorldFramePosition(6)];

%calculate the rotation matrix representing the current orientation
world2Body = quat2rotm(quat);

%matlab issue
world2Body = transpose(world2Body);

== matlab function SMC_mathmatical/SMC/Mathmatical Model/Edot/Target Velocity Gravity Well ==
function targetVelocities = fcn(setPointError, controlParameters)

%the target velocities to converge to - this should always be positive
targetVelocities = zeros(6,1);

controlParametersExpectedLength = 12;
if(~length(controlParameters) == controlParametersExpectedLength)
    %params have not yet been assigned / assgined incorrectly
    return
end

controlParameters = reshape(controlParameters, [length(controlParameters) / 6, 6]);
%param(1,x) = max control value
%param(2,x) = the error where max control is reached

%velocity curves = param(1,x) * (-cos(error * pi / (2 * param(2,x)))^1/2 + 1)
for i=1:6
    if(controlParameters(2, i) == 0 || setPointError(i) == 0)
        targetVelocities(i) = 0;
    else
        %ensure the saturation error is not exceeded
        if(abs(setPointError(i)) > controlParameters(2, i))
            setPointError(i) = controlParameters(2, i) * setPointError(i) / abs(setPointError(i));
        end

        targetVelocities(i) = controlParameters(1,i) * (-abs(cos(setPointError(i) * pi / (2 * controlParameters(2,i))))^(1/2) + 1);
    end


end

== matlab function SMC_mathmatical/SMC/Mathmatical Model/Fm/calculate body frame drag forces ==
function dragForces = fcn(currentBodyVelocities, dragCoefficents)

dragForces = zeros(6,1);

expectedDragCoefficentLength = 24;
if(expectedDragCoefficentLength ~= length(dragCoefficents))
    %drag coefficents are not the expected length
    return 
end

%reshape drag coefficents array into a more sensible form
dc = reshape(dragCoefficents, [expectedDragCoefficentLength / 6, 6]);

for i=1:6
    %calculate the forces created by drag
    dragForces(i) = dc(1, i) + abs(currentBodyVelocities(i)) * dc(2, i) + exp(abs(currentBodyVelocities(i)) / dc(4, i))* dc(3, i);

    %take into account sign
    sign = 0;
    if(currentBodyVelocities(i) ~= 0)
        sign = currentBodyVelocities(i) / abs(currentBodyVelocities(i));
    end

    dragForces(i) = sign * dragForces(i);
end

== matlab function SMC_mathmatical/SMC/Mathmatical Model/Normalize Error ==
function normalizedError = fcn(currentPosition, currentSetPoint)

normalized = zeros(1,6);

normalized(1) = currentPosition(1) - currentSetPoint(1);
normalized(2) = currentPosition(2) - currentSetPoint(2);
normalized(3) = currentPosition(3) - currentSetPoint(3);

W2B = [currentPosition(7), currentPosition(4), currentPosition(5), currentPosition(6)];
setQuat = [currentSetPoint(7), -currentSetPoint(4), -currentSetPoint(5), -currentSetPoint(6)];


%Talos Heading in Body Frame
Tbody = [1,0,0,0];

%Transform from Body 2 World
B2W = [W2B(1), -W2B(2), -W2B(3), -W2B(4)] / (norm(W2B) ^ 2);

%Talos Heading in World Frame
TWorld = quatmultiply(Tbody, B2W);

%Talos Heading in World Frame Conjugate
TWorldI = [TWorld(1), -TWorld(2), -TWorld(3), -TWorld(4)];

%Current Yaw Error
eQuat = quatmultiply(setQuat, TWorldI);

% %axis Error
axisError = [eQuat(2), eQuat(3), eQuat(4)];
if(eQuat(1) < 0)
    axisError = -axisError;
end


normalized(4) = axisError(1);
normalized(5) = axisError(2);
normalized(6) = axisError(3);

normalizedError = normalized;

== matlab function SMC_mathmatical/SMC/Mathmatical Model/S Block/MATLAB Function ==
function [SFlipTime, SSign] = fcn(PreviousSFlipTime, currentError, currentErrorDot, lambda, deltaTime, resetFlipTimeMask)

%FlipTime, SSign and Previous are 6 by arrays - 1 per dof

SFlipTime = PreviousSFlipTime;
SSign = zeros(6,1);

%calculate S
S = currentError + lambda' .* currentErrorDot';


%just so nothing explodes - ill be impressed if this happens
for i=1:6

    %ensure no S equals zero
    if(S(i) == 0)
        SSign(i) = 0;
    else
        SSign(i) = S(i) / abs(S(i));
    end
end


%see if Sdot has flipped
for i=1:6

    %if the flip time is not to be reset
    if(~resetFlipTimeMask(i))
        if(SFlipTime(i) * SSign(i) > 0)
            SFlipTime(i) = SFlipTime(i) + deltaTime * SSign(i);
        else
            SFlipTime(i) = deltaTime * SSign(i);
        end
    else
       SFlipTime(i) = 0;
    end
end
